simulink model "lab2_pogonya2_2018b"  (R2018b)
settings: Solver=FixedStepAuto  StartTime=0.0  StopTime=100  FixedStep=0.05  RelTol=1e-3
libraries: simulink x2
settings Model: Creator=Olya Scherbak  LastModifiedBy=Танечка

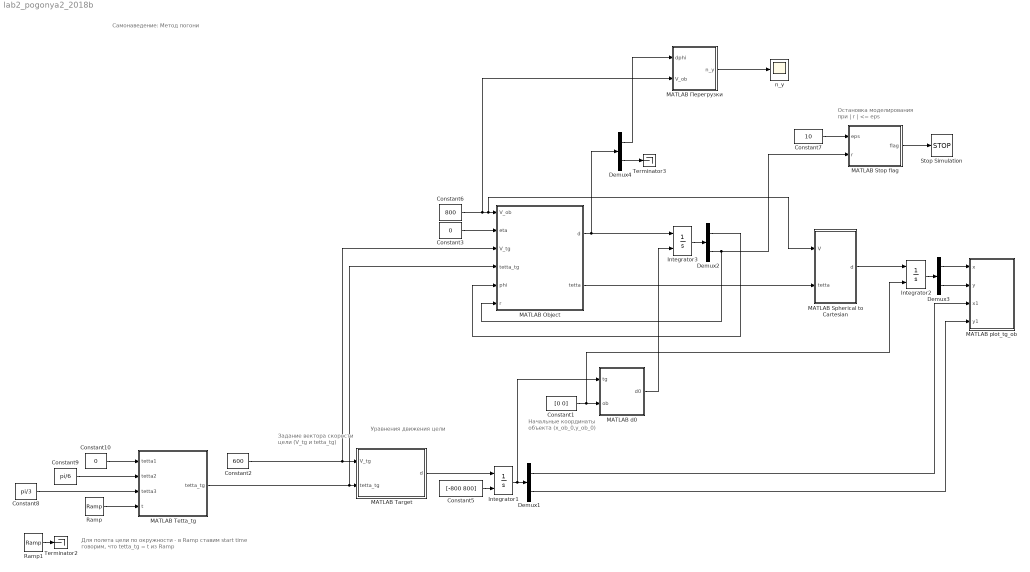
== system lab2_pogonya2_2018b ==
  note: Начальные координаты
      | объекта
      | (x_ob_0,y_ob_0)
  note: Остановка моделирования
      | при | r | <= eps
  note: Задание вектора
      | скорости цели
      | (V_tg и tetta_tg)
  note: Уравнения
      | движения цели
  note: Самонаведение: Метод погони
  note: Для полета цели по окружности - в Ramp ставим start time
      | говорим, что tetta_tg = t из Ramp
  Constant1 : Constant  Value=[0 0]  VectorParams1D=off
  Constant10 : Constant  Value=0
  Constant2 : Constant  Value=600
  Constant3 : Constant  Value=0
  Constant5 : Constant  Value=[-800 800]  VectorParams1D=off
  Constant6 : Constant  Value=800
  Constant7 : Constant  Value=10
  Constant8 : Constant  Value=pi/3
  Constant9 : Constant  Value=pi/6
  Demux{1..4} (4 alike) : Demux  Outputs=2
  Integrator1 : Integrator  InitialConditionSource=external
  Integrator2 : Integrator  InitialConditionSource=external
  Integrator3 : Integrator  InitialConditionSource=external
  MATLAB Object : MATLAB Function  TreatAsAtomicUnit=on
  MATLAB Spherical to Cartesian : MATLAB Function  TreatAsAtomicUnit=on
  MATLAB Stop flag : MATLAB Function  TreatAsAtomicUnit=on
  MATLAB Target : MATLAB Function  TreatAsAtomicUnit=on
  MATLAB Tetta_tg : MATLAB Function  TreatAsAtomicUnit=on
  MATLAB d0 : MATLAB Function  TreatAsAtomicUnit=on
  MATLAB plot_tg_ob : MATLAB Function  TreatAsAtomicUnit=on
  MATLAB Перегрузки : MATLAB Function  TreatAsAtomicUnit=on
  Ramp : simulink/Sources/Ramp  slope=2  start=0  InitialOutput=0
  Ramp1 : simulink/Sources/Ramp  slope=2  start=1.5  InitialOutput=0
  Stop Simulation : Stop
  Terminator2 : Terminator
  Terminator3 : Terminator
  n_y : Scope
  wires:
  MATLAB d0/1(d0) -> Integrator3/2
  Demux2/1 -> MATLAB Object/5(phi)
  MATLAB Tetta_tg/1(tetta_tg) -> MATLAB Object/4(tetta_tg), MATLAB Target/2(tetta_tg)
  MATLAB Object/1(d) -> Integrator3/1, Demux4/1
  MATLAB Перегрузки/1(n_y) -> n_y/1
  Constant2/1 -> MATLAB Object/3(V_tg), MATLAB Target/1(V_tg)
  Demux1/1 -> MATLAB plot_tg_ob/3(x1)
  Integrator3/1 -> Demux2/1
  Demux4/1 -> MATLAB Перегрузки/1(dphi)
  Constant5/1 -> Integrator1/2
  MATLAB Target/1(d) -> Integrator1/1
  Constant7/1 -> MATLAB Stop flag/1(eps)
  Demux2/2 -> MATLAB Stop flag/2(r), MATLAB Object/6(r)
  MATLAB Stop flag/1(flag) -> Stop Simulation/1
  Constant6/1 -> MATLAB Spherical to Cartesian/1(V), MATLAB Object/1(V_ob), MATLAB Перегрузки/2(V_ob)
  Demux1/2 -> MATLAB plot_tg_ob/4(y1)
  MATLAB Spherical to Cartesian/1(d) -> Integrator2/1
  Constant1/1 -> MATLAB d0/2(ob), Integrator2/2
  Integrator1/1 -> MATLAB d0/1(tg), Demux1/1
  Integrator2/1 -> Demux3/1
  Demux3/1 -> MATLAB plot_tg_ob/1(x)
  Demux3/2 -> MATLAB plot_tg_ob/2(y)
  Constant9/1 -> MATLAB Tetta_tg/2(tetta2)
  Constant8/1 -> MATLAB Tetta_tg/3(tetta3)
  Ramp1/1 -> Terminator2/1
  Constant10/1 -> MATLAB Tetta_tg/1(tetta1)
  Ramp/1 -> MATLAB Tetta_tg/4(t)
  Demux4/2 -> Terminator3/1
  MATLAB Object/2(tetta) -> MATLAB Spherical to Cartesian/2(tetta)
  Constant3/1 -> MATLAB Object/2(eta)

== matlab function lab2_pogonya2_2018b/MATLAB Target ==
  data: V_tg input; tetta_tg input; d output
function d   = Target(V_tg, tetta_tg)

% dx = V_tg*t*cos(tetta_tg); 
% dy = V_tg*t*sin(tetta_tg);

dx = V_tg*cos(tetta_tg); 
dy = V_tg*sin(tetta_tg);

d = [dx; dy];

end

== matlab function lab2_pogonya2_2018b/MATLAB d0 ==
  data: tg input; ob input; d0 output
function   d0 = func( tg, ob)

    x = tg(1) - ob(1);
    y = tg(2) - ob(2);

    phi_0 = atan2(y,x); 
    r_0   = sqrt(x^2 + y^2);

    d0 = [phi_0, r_0];

end

== matlab function lab2_pogonya2_2018b/MATLAB Перегрузки ==
  data: dphi input; V_ob input; n_y output
function n_y  = func( dphi,V_ob)

g = 9.81;

n_y = V_ob*dphi/g;


end

== matlab function lab2_pogonya2_2018b/MATLAB Tetta_tg ==
  data: tetta1 input; tetta2 input; tetta3 input; tetta_tg output; t input
function tetta_tg   = Target(tetta1, tetta2, tetta3, t)

tetta_tg = tetta1;

if (t>=0)&&(t<=0.8)
    tetta_tg = tetta1;
end
if (t>0.8)&&(t<=1.5)
    tetta_tg = tetta2;
end
if t>1.2
    tetta_tg = tetta3;
end
% tetta_tg = t;

end

== matlab function lab2_pogonya2_2018b/MATLAB Object ==
  data: d output; V_ob input; eta input; V_tg input; tetta_tg input; phi input; r input; tetta output
function [d, tetta]  = Object(V_ob, eta, V_tg, tetta_tg, phi, r)

    tetta = phi - eta;
    dr    =  -V_ob*cos(phi - tetta) + V_tg*cos(phi - tetta_tg);
    dphi  =  (V_ob*sin(phi - tetta))/r - (V_tg*sin(phi - tetta_tg))/r;
   
    d = [dphi; dr];
end

== matlab function lab2_pogonya2_2018b/MATLAB Spherical to Cartesian ==
  data: V input; tetta input; d output
function d = func(V, tetta)

% Из сферической системе координат в декартову

    dx = V*cos(tetta);
    dy = V*sin(tetta);             

    d = [dx, dy];

end

== matlab function lab2_pogonya2_2018b/MATLAB plot_tg_ob ==
  data: x input; y input; x1 input; y1 input
function plot2d(x,y, x1, y1)

figure(3);
plot(x,y,'ob');
hold on;
plot(x1,y1,'or');
hold on;

xlabel('X');
ylabel('Y');


grid on;
grid minor;
axis('equal');
end

== matlab function lab2_pogonya2_2018b/MATLAB Stop flag ==
  data: eps input; r input; flag output
function flag  = Stop_flag(eps, r)

flag = 0;

if abs(r) < eps
          flag = 1;          
end
     
end
